simulink model "sway_linear"  (R2020a)
settings: Solver=VariableStepAuto  StartTime=0.0  StopTime=500  RelTol=1e-3
settings Model: Creator=xiaoran  LastModifiedBy=xiaoran

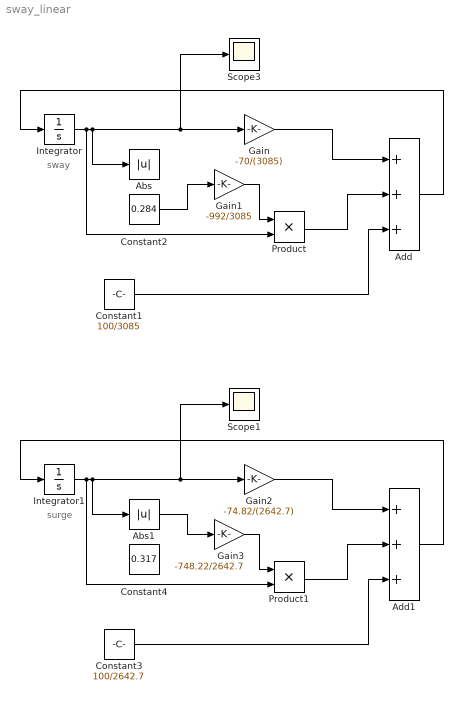
== system sway_linear ==
  note: sway
  note: surge
  Abs : Abs
  Abs1 : Abs
  Add : Sum  Inputs=+++
  Add1 : Sum  Inputs=+++
  Constant1 : Constant  Value=100/3085
  Constant2 : Constant  Value=0.284
  Constant3 : Constant  Value=100/2642.7
  Constant4 : Constant  Value=0.317
  Gain : Gain  Gain=-70/(3085)
  Gain1 : Gain  Gain=-992/3085
  Gain2 : Gain  Gain=-74.82/(2642.7)
  Gain3 : Gain  Gain=-748.22/2642.7
  Integrator : Integrator  InitialCondition=.1
  Integrator1 : Integrator  InitialCondition=.1
  Product : Product
  Product1 : Product
  Scope1 : Scope
  Scope3 : Scope
  wires:
  Integrator/1 -> Product/2, Abs/1, Scope3/1, Gain/1
  Gain1/1 -> Product/1
  Gain/1 -> Add/1
  Product/1 -> Add/2
  Constant1/1 -> Add/3
  Add/1 -> Integrator/1
  Constant2/1 -> Gain1/1
  Add1/1 -> Integrator1/1
  Constant3/1 -> Add1/3
  Product1/1 -> Add1/2
  Gain2/1 -> Add1/1
  Gain3/1 -> Product1/1
  Integrator1/1 -> Gain2/1, Scope1/1, Abs1/1, Product1/2
  Abs1/1 -> Gain3/1
